simulink model "practica3"  (R2019b)
settings: Solver=FixedStepAuto  StartTime=0.0  StopTime=10.0  RelTol=1e-3  EnableMultiTasking=on
undefined symbols (not defined in the file): t_sim
libraries: legoev3lib x3, simulink x1
settings Model: ExtModeTrigDuration=2  Creator=alumnopr09  LastModifiedBy=alumnopr09
settings SolverCC: PositivePriorityOrder=on
settings OptimizationCC: EnhancedBackFolding=on  PassReuseOutputArgsAs=Individual arguments  ZeroExternalMemoryAtStartup=off  ZeroInternalMemoryAtStartup=off  MaxStackSize=64  OptimizeBlockOrder=speed  DifferentSizesBufferReuse=on  OptimizationCustomize=off  EfficientTunableParamExpr=on
settings DebuggingCC: ParameterTunabilityLossMsg=error
settings HardwareCC: ProdBitPerPointer=32  ProdBitPerSizeT=32  ProdBitPerPtrDiffT=32  ProdLargestAtomicInteger=Long  ProdWordSize=32  ProdHWDeviceType=ARM Compatible->ARM 9
settings SFSimCC: MATLABDynamicMemAlloc=off
settings RTWCC: SystemTargetFile=ert.tlc  HardwareBoard=LEGO MINDSTORMS EV3  TLCOptions="-aInlineSetEventsForThisBaseRateFcn=TLC_FALSE -aSuppressMultiTaskScheduler=TLC_FALSE  -aRateBasedStepFcn=0"  TemplateMakefile=ert_default_tmf  GenerateReport=on  Toolchain=Sourcery G++ Lite v2009q3  IncludeHyperlinkInReport=on  LaunchReport=on  GenerateTraceInfo=on  GenerateTraceReport=on  GenerateTraceReportSl=on  GenerateTraceReportSf=on  GenerateTraceReportEml=on
settings CodeAppCC: ForceParamTrailComments=on  IgnoreCustomStorageClasses=off  OperatorAnnotations=on  SimulinkDataObjDesc=on  SFDataObjDesc=on  InsertBlockDesc=on
settings ERTTargetCC: SupportContinuousTime=on  SupportVariableSizeSignals=on

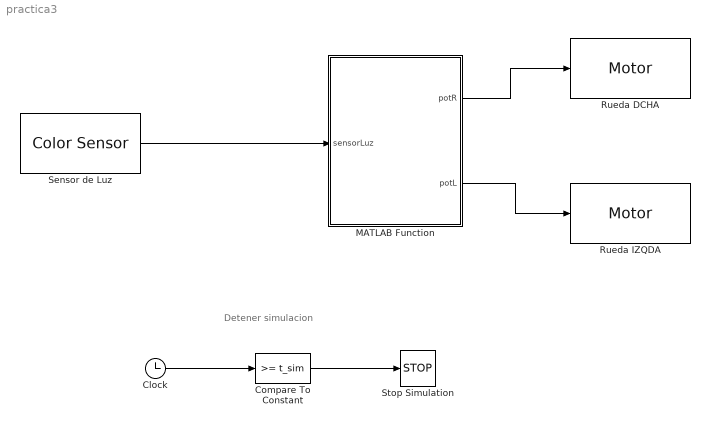
== system practica3 ==
  note: Detener simulacion
  Clock : Clock
  Compare To Constant : simulink/Logic and Bit Operations/Compare To Constant  relop=>=  const=t_sim  OutDataTypeStr=boolean
  MATLAB Function : MATLAB Function  TreatAsAtomicUnit=on
  Rueda DCHA : legoev3lib/Motor  sportNumber=C  sstopAction=Brake
  Rueda IZQDA : legoev3lib/Motor  sportNumber=B  sstopAction=Brake
  Sensor de Luz : legoev3lib/Color Sensor  portNumber=4  mode=Reflected light intensity  sampleTime=0.1
      settings: SourceProductName=Simulink Support Package for LEGO MINDSTORMS EV3 Hardware  SourceProductBaseCode=LEGOEV3
  Stop Simulation : Stop
  wires:
  Compare To Constant/1 -> Stop Simulation/1
  Clock/1 -> Compare To Constant/1
  Sensor de Luz/1 -> MATLAB Function/1(sensorLuz)
  MATLAB Function/1(potR) -> Rueda DCHA/1
  MATLAB Function/2(potL) -> Rueda IZQDA/1

== matlab function practica3/MATLAB Function ==
  data: sensorLuz input; potR output; potL output
function [potR, potL] = fcn(sensorLuz)
    % Constantes generales
    Kp = 0.5;
    Ki = 0.05;
    Kd = 0.1;
    BLANCO = 70;
    NEGRO = 35;
    P = 10;
   
    % Inicializacion de variables
    sat = 60;
    wup = 30;
    
    persistent integral;
    if (isempty(integral))
        integral= 0;
    end
    
    persistent lastError;
    if (isempty(lastError))
        lastError = 0;
    end
    
    % Calibracion de luz del sensor
    blanco = 69;
    negro = 6;

    % Lectura del sensor
    sensorLuz_d = double(sensorLuz);
    % Ajuste de lectura a los niveles del sensor
    lightValue = (sensorLuz_d*(BLANCO-NEGRO)/(blanco-negro))+((-negro*(BLANCO-NEGRO))+(NEGRO*(blanco-negro)))/(blanco-negro);
    error = lightValue - (BLANCO+NEGRO)/2;
    integral = integral + error;
    derivate = error - lastError;
    % Actualizacion de la actuacion del controlador
    turn = Kp*error + Ki*integral + Kd*derivate;
    % Ajuste de actuacion con WIND-UP
    if (turn > wup)
        turn =  Kp*error + Kd*derivate;
        integral = integral - error;
    end

    potR = P + turn;
    potL = P - turn;
    % Ajuste de la potencia de los motores con sat.
    if (potR > sat)
        potR = sat;
    end
    if (potL > sat)
        potL = -sat;
    end
    lastError = error;
